simulink model "RLFactorySensorNoise"  (R2020b)
settings: Solver=VariableStepAuto  StartTime=0.0  StopTime=10.0  RelTol=1e-3
undefined symbols (not defined in the file): BLOCKEDTIMER, CUTOFF, DMAX, GOALSA, GOALSB, INITBX, INITBY, INTERFERENCEMAX, INTERFERENCEMIN, MAXVELOA, MAXVELOB, SAFETYDISTANCEA, SAFETYDISTANCEB, THRESHOLDA, THRESHOLDB, TSA, TSB, TSRL
libraries: rllib x1
(part 1 of 2)
settings Model: Creator=julius  LastModifiedBy=julius

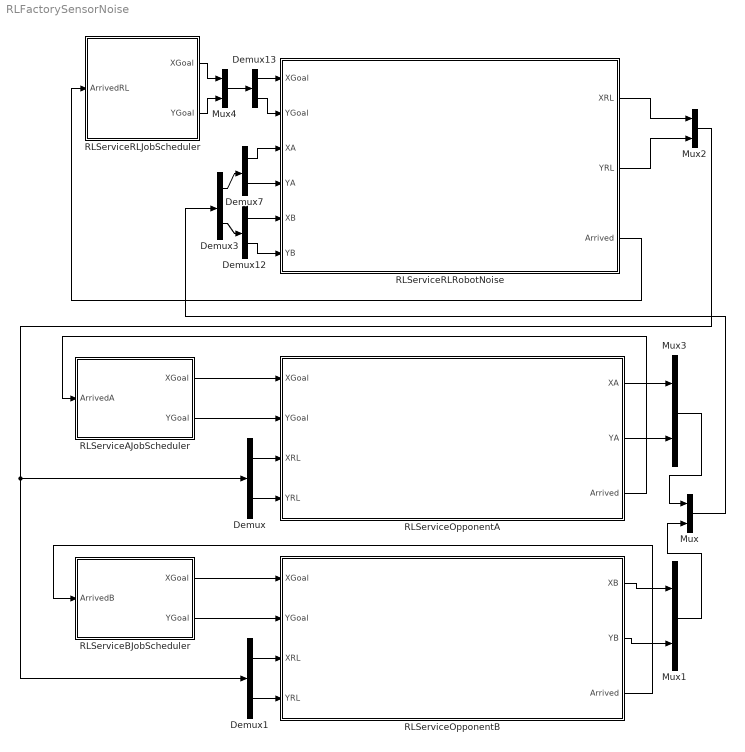
== system RLFactorySensorNoise ==
  Demux{,1,3,7,12..13} (6 alike) : Demux  Outputs=2
  Mux{,1..4} (5 alike) : Mux  Inputs=2
  RLServiceAJobScheduler : Subsystem
  RLServiceBJobScheduler : Subsystem
  RLServiceOpponentA : Subsystem
  RLServiceOpponentB : Subsystem
  RLServiceRLJobScheduler : Subsystem
  RLServiceRLRobotNoise : Subsystem
  wires:
  RLServiceRLJobScheduler/2(YGoal) -> Mux4/2
  RLServiceRLJobScheduler/1(XGoal) -> Mux4/1
  Mux4/1 -> Demux13/1
  Demux3/1 -> Demux7/1
  Demux3/2 -> Demux12/1
  Demux13/1 -> RLServiceRLRobotNoise/1(XGoal)
  Demux13/2 -> RLServiceRLRobotNoise/2(YGoal)
  Demux7/1 -> RLServiceRLRobotNoise/3(XA)
  Demux7/2 -> RLServiceRLRobotNoise/4(YA)
  Demux12/1 -> RLServiceRLRobotNoise/5(XB)
  Demux12/2 -> RLServiceRLRobotNoise/6(YB)
  RLServiceRLRobotNoise/3(Arrived) -> RLServiceRLJobScheduler/1(ArrivedRL)
  RLServiceRLRobotNoise/1(XRL) -> Mux2/1
  RLServiceRLRobotNoise/2(YRL) -> Mux2/2
  RLServiceOpponentB/3(Arrived) -> RLServiceBJobScheduler/1(ArrivedB)
  Demux1/2 -> RLServiceOpponentB/4(YRL)
  Demux/2 -> RLServiceOpponentA/4(YRL)
  Mux1/1 -> Mux/2
  RLServiceBJobScheduler/2(YGoal) -> RLServiceOpponentB/2(YGoal)
  RLServiceBJobScheduler/1(XGoal) -> RLServiceOpponentB/1(XGoal)
  RLServiceOpponentA/1(XA) -> Mux3/1
  RLServiceOpponentB/1(XB) -> Mux1/1
  Demux1/1 -> RLServiceOpponentB/3(XRL)
  Mux/1 -> Demux3/1
  RLServiceOpponentB/2(YB) -> Mux1/2
  RLServiceOpponentA/2(YA) -> Mux3/2
  RLServiceAJobScheduler/2(YGoal) -> RLServiceOpponentA/2(YGoal)
  RLServiceOpponentA/3(Arrived) -> RLServiceAJobScheduler/1(ArrivedA)
  Demux/1 -> RLServiceOpponentA/3(XRL)
  RLServiceAJobScheduler/1(XGoal) -> RLServiceOpponentA/1(XGoal)
  Mux3/1 -> Mux/1
  Mux2/1 -> Demux1/1, Demux/1

== system RLFactorySensorNoise/RLServiceAJobScheduler ==
  ArrivedA : Inport
  Constant1 : Constant  Value=GOALSA
  JobScheduler2 : MATLABSystem  System=JobScheduler  SimulateUsing=Interpreted execution
      mask Type: JobScheduler
      mask Display:
      | disp('JobScheduler');
      | port_label('input',1,'workstations');
      | port_label('input',2,'done');
      | port_label('output',1,'currentGoalX');
      | port_label('output',2,'currentGoalY');
  XGoal : Outport
  YGoal : Outport  Port=2
  wires:
  Constant1/1 -> JobScheduler2/1
  JobScheduler2/2 -> YGoal/1
  ArrivedA/1 -> JobScheduler2/2
  JobScheduler2/1 -> XGoal/1

== system RLFactorySensorNoise/RLServiceBJobScheduler ==
  ArrivedB : Inport
  Constant1 : Constant  Value=GOALSB
  JobScheduler2 : MATLABSystem  System=JobScheduler  SimulateUsing=Interpreted execution
      mask Type: JobScheduler
      mask Display:
      | disp('JobScheduler');
      | port_label('input',1,'workstations');
      | port_label('input',2,'done');
      | port_label('output',1,'currentGoalX');
      | port_label('output',2,'currentGoalY');
  XGoal : Outport
  YGoal : Outport  Port=2
  wires:
  Constant1/1 -> JobScheduler2/1
  JobScheduler2/2 -> YGoal/1
  ArrivedB/1 -> JobScheduler2/2
  JobScheduler2/1 -> XGoal/1

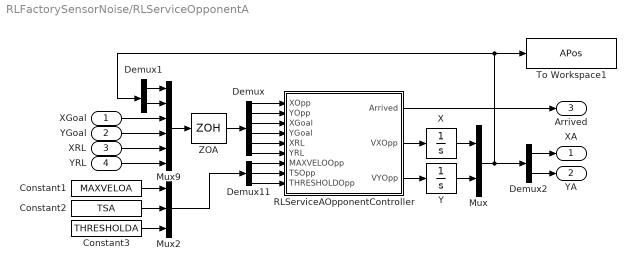
== system RLFactorySensorNoise/RLServiceOpponentA ==
  XGoal : Inport
  YGoal : Inport  Port=2
  XRL : Inport  Port=3
  YRL : Inport  Port=4
  Constant1 : Constant  Value=MAXVELOA
  Constant2 : Constant  Value=TSA
  Constant3 : Constant  Value=THRESHOLDA
  Demux : Demux  Outputs=6
  Demux1 : Demux  Outputs=2
  Demux11 : Demux  Outputs=3
  Demux2 : Demux  Outputs=2
  Mux : Mux  Inputs=2
  Mux2 : Mux  Inputs=3
  Mux9 : Mux  Inputs=6
  RLServiceAOpponentController : Subsystem
  To Workspace1 : ToWorkspace  VariableName=APos  SampleTime=0.25
  X : Integrator  InitialCondition=5
  Y : Integrator  InitialCondition=5
  ZOA : ZeroOrderHold  SampleTime=TSA
  XA : Outport
  YA : Outport  Port=2
  Arrived : Outport  Port=3
  wires:
  RLServiceAOpponentController/1(Arrived) -> Arrived/1
  Demux/4 -> RLServiceAOpponentController/4(YGoal)
  Demux/6 -> RLServiceAOpponentController/6(YRL)
  X/1 -> Mux/1
  YRL/1 -> Mux9/6
  Demux/5 -> RLServiceAOpponentController/5(XRL)
  YGoal/1 -> Mux9/4
  Demux/1 -> RLServiceAOpponentController/1(XOpp)
  Y/1 -> Mux/2
  Mux/1 -> Demux1/1, To Workspace1/1, Demux2/1
  Mux9/1 -> ZOA/1
  Demux/3 -> RLServiceAOpponentController/3(XGoal)
  Demux/2 -> RLServiceAOpponentController/2(YOpp)
  XRL/1 -> Mux9/5
  ZOA/1 -> Demux/1
  XGoal/1 -> Mux9/3
  Mux2/1 -> Demux11/1
  Demux1/1 -> Mux9/1
  Demux1/2 -> Mux9/2
  Constant2/1 -> Mux2/2
  Constant1/1 -> Mux2/1
  Constant3/1 -> Mux2/3
  Demux2/1 -> XA/1
  Demux2/2 -> YA/1
  RLServiceAOpponentController/3(VYOpp) -> Y/1
  RLServiceAOpponentController/2(VXOpp) -> X/1
  Demux11/1 -> RLServiceAOpponentController/7(MAXVELOOpp)
  Demux11/2 -> RLServiceAOpponentController/8(TSOpp)
  Demux11/3 -> RLServiceAOpponentController/9(THRESHOLDOpp)

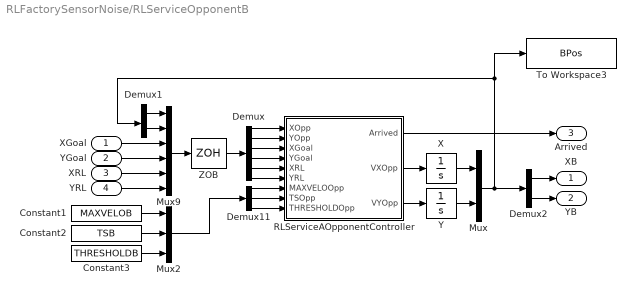
== system RLFactorySensorNoise/RLServiceOpponentB ==
  XGoal : Inport
  YGoal : Inport  Port=2
  XRL : Inport  Port=3
  YRL : Inport  Port=4
  Constant1 : Constant  Value=MAXVELOB
  Constant2 : Constant  Value=TSB
  Constant3 : Constant  Value=THRESHOLDB
  Demux : Demux  Outputs=6
  Demux1 : Demux  Outputs=2
  Demux11 : Demux  Outputs=3
  Demux2 : Demux  Outputs=2
  Mux : Mux  Inputs=2
  Mux2 : Mux  Inputs=3
  Mux9 : Mux  Inputs=6
  RLServiceAOpponentController : Subsystem
  To Workspace3 : ToWorkspace  VariableName=BPos  SampleTime=0.25
  X : Integrator  InitialCondition=randi(INITBX)
  Y : Integrator  InitialCondition=randi(INITBY)
  ZOB : ZeroOrderHold  SampleTime=TSB
  XB : Outport
  YB : Outport  Port=2
  Arrived : Outport  Port=3
  wires:
  RLServiceAOpponentController/3(VYOpp) -> Y/1
  XRL/1 -> Mux9/5
  Demux11/1 -> RLServiceAOpponentController/7(MAXVELOOpp)
  Constant2/1 -> Mux2/2
  RLServiceAOpponentController/2(VXOpp) -> X/1
  Mux9/1 -> ZOB/1
  Constant3/1 -> Mux2/3
  Demux1/2 -> Mux9/2
  Demux/1 -> RLServiceAOpponentController/1(XOpp)
  YGoal/1 -> Mux9/4
  Demux/4 -> RLServiceAOpponentController/4(YGoal)
  RLServiceAOpponentController/1(Arrived) -> Arrived/1
  X/1 -> Mux/1
  Mux/1 -> To Workspace3/1, Demux1/1, Demux2/1
  Demux/6 -> RLServiceAOpponentController/6(YRL)
  Demux/3 -> RLServiceAOpponentController/3(XGoal)
  Demux1/1 -> Mux9/1
  Demux11/2 -> RLServiceAOpponentController/8(TSOpp)
  Demux2/1 -> XB/1
  YRL/1 -> Mux9/6
  Demux/2 -> RLServiceAOpponentController/2(YOpp)
  Demux11/3 -> RLServiceAOpponentController/9(THRESHOLDOpp)
  ZOB/1 -> Demux/1
  Demux2/2 -> YB/1
  Mux2/1 -> Demux11/1
  Constant1/1 -> Mux2/1
  XGoal/1 -> Mux9/3
  Y/1 -> Mux/2
  Demux/5 -> RLServiceAOpponentController/5(XRL)

== system RLFactorySensorNoise/RLServiceRLJobScheduler ==
  ArrivedRL : Inport
  Constant : Constant  Value=[[-3;4],[5;5],[-5;-5],[5;2]]
  JobScheduler1 : MATLABSystem  System=JobScheduler  SimulateUsing=Interpreted execution
      mask Type: JobScheduler
      mask Display:
      | disp('JobScheduler');
      | port_label('input',1,'workstations');
      | port_label('input',2,'done');
      | port_label('output',1,'currentGoalX');
      | port_label('output',2,'currentGoalY');
  Mux2 : Mux  Inputs=2
  To Workspace2 : ToWorkspace  VariableName=Job  SampleTime=0.25
  XGoal : Outport
  YGoal : Outport  Port=2
  wires:
  Constant/1 -> JobScheduler1/1
  JobScheduler1/2 -> Mux2/2, YGoal/1
  ArrivedRL/1 -> JobScheduler1/2
  JobScheduler1/1 -> Mux2/1, XGoal/1
  Mux2/1 -> To Workspace2/1

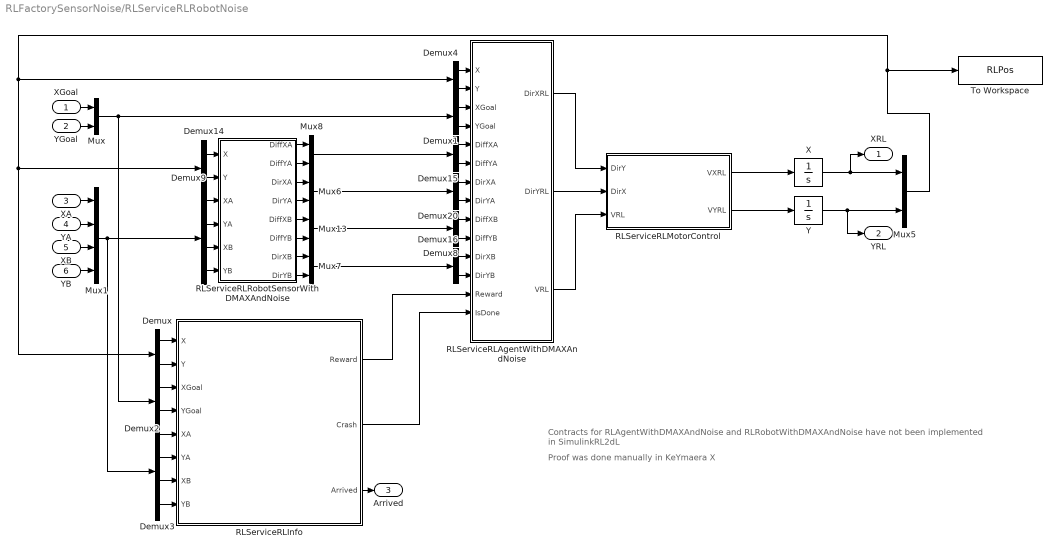
== system RLFactorySensorNoise/RLServiceRLRobotNoise ==
  note: Proof was done manually in KeYmaera X
  note: Contracts for RLAgentWithDMAXAndNoise and RLRobotWithDMAXAndNoise have not been implemented in SimulinkRL2dL
  XGoal : Inport
  YGoal : Inport  Port=2
  XA : Inport  Port=3
  YA : Inport  Port=4
  XB : Inport  Port=5
  YB : Inport  Port=6
  Demux{,1..2,4,8,14..16,20} (9 alike) : Demux  Outputs=2
  Demux3 : Demux
  Demux9 : Demux
  Mux{,5..8,13} (6 alike) : Mux  Inputs=2
  Mux1 : Mux
  RLServiceRLAgentWithDMAXAndNoise : Subsystem
  RLServiceRLInfo : Subsystem
  RLServiceRLMotorControl : Subsystem
  RLServiceRLRobotSensorWithDMAXAndNoise : Subsystem
  To Workspace : ToWorkspace  VariableName=RLPos  SampleTime=0.25
  X : Integrator  InitialCondition=-3
  Y : Integrator  InitialCondition=-5
  XRL : Outport
  YRL : Outport  Port=2
  Arrived : Outport  Port=3
  wires:
  XA/1 -> Mux1/1
  X/1 -> Mux5/1, XRL/1
  Mux13/1 -> Demux8/1
  Demux4/1 -> RLServiceRLAgentWithDMAXAndNoise/1(X)
  RLServiceRLRobotSensorWithDMAXAndNoise/5(DiffXB) -> Mux13/1
  Demux4/2 -> RLServiceRLAgentWithDMAXAndNoise/2(Y)
  Demux14/2 -> RLServiceRLRobotSensorWithDMAXAndNoise/2(Y)
  Demux15/1 -> RLServiceRLAgentWithDMAXAndNoise/5(DiffXA)
  RLServiceRLRobotSensorWithDMAXAndNoise/4(DirYA) -> Mux6/2
  XGoal/1 -> Mux/1
  Demux20/2 -> RLServiceRLAgentWithDMAXAndNoise/8(DirYA)
  RLServiceRLRobotSensorWithDMAXAndNoise/2(DiffYA) -> Mux8/2
  RLServiceRLRobotSensorWithDMAXAndNoise/7(DirXB) -> Mux7/1
  Mux/1 -> Demux2/1, Demux1/1
  Demux1/2 -> RLServiceRLAgentWithDMAXAndNoise/4(YGoal)
  Demux16/1 -> RLServiceRLAgentWithDMAXAndNoise/11(DirXB)
  RLServiceRLInfo/1(Reward) -> RLServiceRLAgentWithDMAXAndNoise/13(Reward)
  Demux15/2 -> RLServiceRLAgentWithDMAXAndNoise/6(DiffYA)
  Demux1/1 -> RLServiceRLAgentWithDMAXAndNoise/3(XGoal)
  Y/1 -> YRL/1, Mux5/2
  RLServiceRLRobotSensorWithDMAXAndNoise/3(DirXA) -> Mux6/1
  RLServiceRLAgentWithDMAXAndNoise/2(DirYRL) -> RLServiceRLMotorControl/2(DirX)
  Mux1/1 -> Demux3/1, Demux9/1
  Demux20/1 -> RLServiceRLAgentWithDMAXAndNoise/7(DirXA)
  RLServiceRLRobotSensorWithDMAXAndNoise/8(DirYB) -> Mux7/2
  Demux8/1 -> RLServiceRLAgentWithDMAXAndNoise/9(DiffXB)
  YB/1 -> Mux1/4
  YGoal/1 -> Mux/2
  Mux5/1 -> Demux4/1, Demux/1, Demux14/1, To Workspace/1
  Mux6/1 -> Demux20/1
  RLServiceRLAgentWithDMAXAndNoise/1(DirXRL) -> RLServiceRLMotorControl/1(DirY)
  RLServiceRLRobotSensorWithDMAXAndNoise/1(DiffXA) -> Mux8/1
  Mux7/1 -> Demux16/1
  XB/1 -> Mux1/3
  Demux16/2 -> RLServiceRLAgentWithDMAXAndNoise/12(DirYB)
  YA/1 -> Mux1/2
  Demux8/2 -> RLServiceRLAgentWithDMAXAndNoise/10(DiffYB)
  Mux8/1 -> Demux15/1
  Demux14/1 -> RLServiceRLRobotSensorWithDMAXAndNoise/1(X)
  RLServiceRLRobotSensorWithDMAXAndNoise/6(DiffYB) -> Mux13/2
  RLServiceRLAgentWithDMAXAndNoise/3(VRL) -> RLServiceRLMotorControl/3(VRL)
  RLServiceRLMotorControl/1(VXRL) -> X/1
  RLServiceRLMotorControl/2(VYRL) -> Y/1
  RLServiceRLInfo/2(Crash) -> RLServiceRLAgentWithDMAXAndNoise/14(IsDone)
  RLServiceRLInfo/3(Arrived) -> Arrived/1
  Demux9/1 -> RLServiceRLRobotSensorWithDMAXAndNoise/3(XA)
  Demux9/2 -> RLServiceRLRobotSensorWithDMAXAndNoise/4(YA)
  Demux9/3 -> RLServiceRLRobotSensorWithDMAXAndNoise/5(XB)
  Demux9/4 -> RLServiceRLRobotSensorWithDMAXAndNoise/6(YB)
  Demux/1 -> RLServiceRLInfo/1(X)
  Demux/2 -> RLServiceRLInfo/2(Y)
  Demux2/1 -> RLServiceRLInfo/3(XGoal)
  Demux2/2 -> RLServiceRLInfo/4(YGoal)
  Demux3/1 -> RLServiceRLInfo/5(XA)
  Demux3/2 -> RLServiceRLInfo/6(YA)
  Demux3/3 -> RLServiceRLInfo/7(XB)
  Demux3/4 -> RLServiceRLInfo/8(YB)

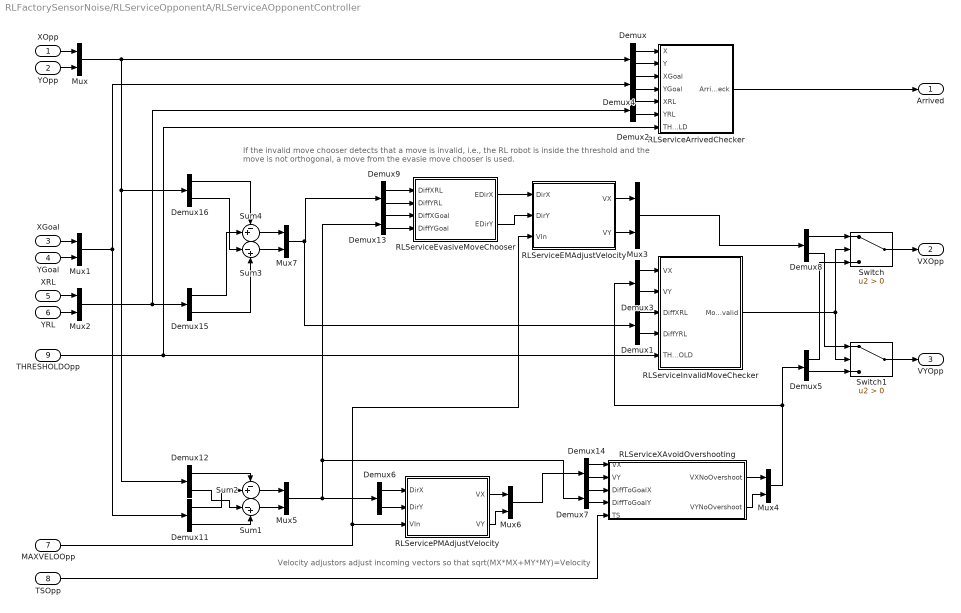
== system RLFactorySensorNoise/RLServiceOpponentA/RLServiceAOpponentController ==
  note: If the invalid move chooser detects that a move is invalid, i.e.,
      | the RL robot is inside the threshold and the move is not orthogonal, a move from the evasie move chooser is used.
  note: Velocity adjustors adjust incoming vectors so that sqrt(MX*MX+MY*MY)=Velocity
  XOpp : Inport
  YOpp : Inport  Port=2
  XGoal : Inport  Port=3
  YGoal : Inport  Port=4
  XRL : Inport  Port=5
  YRL : Inport  Port=6
  MAXVELOOpp : Inport  Port=7
  TSOpp : Inport  Port=8
  THRESHOLDOpp : Inport  Port=9
  Demux{,1..9,11..16} (16 alike) : Demux  Outputs=2
  Mux{,1..7} (8 alike) : Mux  Inputs=2
  RLServiceArrivedChecker : Subsystem
  RLServiceEMAdjustVelocity : Subsystem
  RLServiceEvasiveMoveChooser : Subsystem
  RLServiceInvalidMoveChecker : Subsystem
  RLServicePMAdjustVelocity : Subsystem
  RLServiceXAvoidOvershooting : Subsystem
  Sum1 : Sum  Inputs=|-+
  Sum2 : Sum  Inputs=-+|
  Sum3 : Sum  Inputs=|-+
  Sum4 : Sum  Inputs=-+|
  Switch : Switch  Criteria=u2 > Threshold
  Switch1 : Switch  Criteria=u2 > Threshold
  Arrived : Outport
  VXOpp : Outport  Port=2
  VYOpp : Outport  Port=3
  wires:
  XGoal/1 -> Mux1/1
  YGoal/1 -> Mux1/2
  RLServiceArrivedChecker/1(ArrivedCheck) -> Arrived/1
  Demux/1 -> RLServiceArrivedChecker/1(X)
  Demux/2 -> RLServiceArrivedChecker/2(Y)
  Demux4/1 -> RLServiceArrivedChecker/3(XGoal)
  Demux4/2 -> RLServiceArrivedChecker/4(YGoal)
  XOpp/1 -> Mux/1
  YOpp/1 -> Mux/2
  XRL/1 -> Mux2/1
  YRL/1 -> Mux2/2
  Demux3/1 -> RLServiceInvalidMoveChecker/1(VX)
  Demux8/1 -> Switch/1
  Demux5/2 -> Switch1/3
  Demux8/2 -> Switch1/1
  THRESHOLDOpp/1 -> RLServiceArrivedChecker/7(THRESHOLD), RLServiceInvalidMoveChecker/5(THRESHOLD)
  Demux3/2 -> RLServiceInvalidMoveChecker/2(VY)
  Demux5/1 -> Switch/3
  RLServiceInvalidMoveChecker/1(MoveInvalid) -> Switch/2, Switch1/2
  Switch/1 -> VXOpp/1
  Switch1/1 -> VYOpp/1
  Mux5/1 -> Demux6/1, Demux7/1, Demux13/1
  Demux6/2 -> RLServicePMAdjustVelocity/2(DirY)
  Mux1/1 -> Demux4/1, Demux11/1
  TSOpp/1 -> RLServiceXAvoidOvershooting/5(TS)
  MAXVELOOpp/1 -> RLServiceEMAdjustVelocity/3(VIn), RLServicePMAdjustVelocity/3(VIn)
  RLServicePMAdjustVelocity/1(VX) -> Mux6/1
  RLServicePMAdjustVelocity/2(VY) -> Mux6/2
  RLServiceEvasiveMoveChooser/1(EDirX) -> RLServiceEMAdjustVelocity/1(DirX)
  RLServiceEvasiveMoveChooser/2(EDirY) -> RLServiceEMAdjustVelocity/2(DirY)
  RLServiceEMAdjustVelocity/1(VX) -> Mux3/1
  RLServiceEMAdjustVelocity/2(VY) -> Mux3/2
  Mux3/1 -> Demux8/1
  RLServiceXAvoidOvershooting/1(VXNoOvershoot) -> Mux4/1
  RLServiceXAvoidOvershooting/2(VYNoOvershoot) -> Mux4/2
  Mux4/1 -> Demux5/1, Demux3/1
  Sum2/1 -> Mux5/1
  Sum1/1 -> Mux5/2
  Demux6/1 -> RLServicePMAdjustVelocity/1(DirX)
  Demux7/1 -> RLServiceXAvoidOvershooting/3(DiffToGoalX)
  Demux7/2 -> RLServiceXAvoidOvershooting/4(DiffToGoalY)
  Demux13/1 -> RLServiceEvasiveMoveChooser/3(DiffXGoal)
  Demux13/2 -> RLServiceEvasiveMoveChooser/4(DiffYGoal)
  Demux11/1 -> Sum2/2
  Demux12/2 -> Sum1/1
  Demux11/2 -> Sum1/2
  Demux12/1 -> Sum2/1
  Demux14/1 -> RLServiceXAvoidOvershooting/1(VX)
  Demux14/2 -> RLServiceXAvoidOvershooting/2(VY)
  Mux6/1 -> Demux14/1
  Sum3/1 -> Mux7/2
  Demux16/1 -> Sum4/1
  Sum4/1 -> Mux7/1
  Mux/1 -> Demux12/1, Demux16/1, Demux/1
  Mux2/1 -> Demux2/1, Demux15/1
  Demux15/2 -> Sum3/2
  Demux15/1 -> Sum4/2
  Demux16/2 -> Sum3/1
  Demux9/1 -> RLServiceEvasiveMoveChooser/1(DiffXRL)
  Demux9/2 -> RLServiceEvasiveMoveChooser/2(DiffYRL)
  Mux7/1 -> Demux1/1, Demux9/1
  Demux1/1 -> RLServiceInvalidMoveChecker/3(DiffXRL)
  Demux1/2 -> RLServiceInvalidMoveChecker/4(DiffYRL)
  Demux2/2 -> RLServiceArrivedChecker/6(YRL)
  Demux2/1 -> RLServiceArrivedChecker/5(XRL)

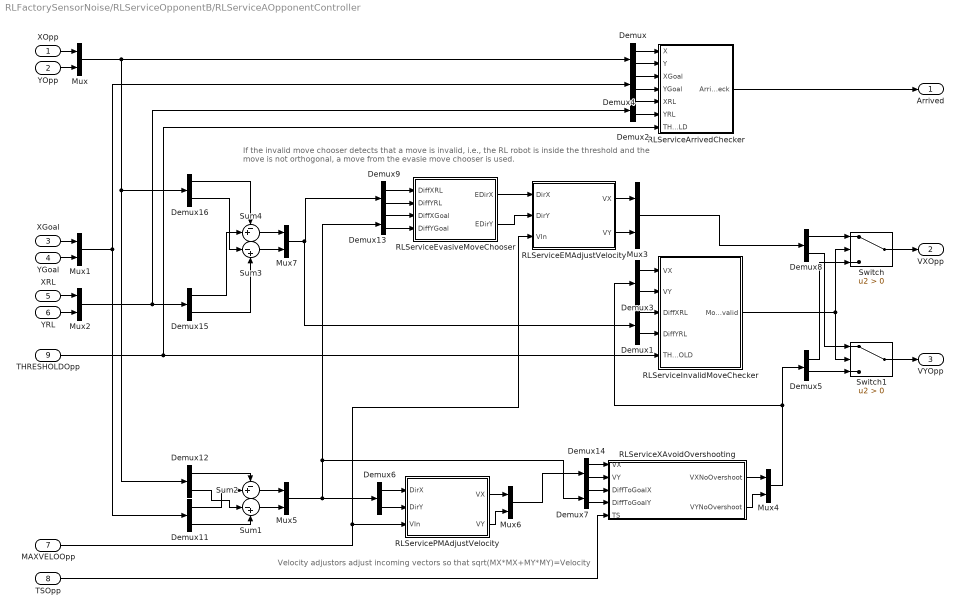
== system RLFactorySensorNoise/RLServiceOpponentB/RLServiceAOpponentController ==
  note: If the invalid move chooser detects that a move is invalid, i.e.,
      | the RL robot is inside the threshold and the move is not orthogonal, a move from the evasie move chooser is used.
  note: Velocity adjustors adjust incoming vectors so that sqrt(MX*MX+MY*MY)=Velocity
  XOpp : Inport
  YOpp : Inport  Port=2
  XGoal : Inport  Port=3
  YGoal : Inport  Port=4
  XRL : Inport  Port=5
  YRL : Inport  Port=6
  MAXVELOOpp : Inport  Port=7
  TSOpp : Inport  Port=8
  THRESHOLDOpp : Inport  Port=9
  Demux{,1..9,11..16} (16 alike) : Demux  Outputs=2
  Mux{,1..7} (8 alike) : Mux  Inputs=2
  RLServiceArrivedChecker : Subsystem
  RLServiceEMAdjustVelocity : Subsystem
  RLServiceEvasiveMoveChooser : Subsystem
  RLServiceInvalidMoveChecker : Subsystem
  RLServicePMAdjustVelocity : Subsystem
  RLServiceXAvoidOvershooting : Subsystem
  Sum1 : Sum  Inputs=|-+
  Sum2 : Sum  Inputs=-+|
  Sum3 : Sum  Inputs=|-+
  Sum4 : Sum  Inputs=-+|
  Switch : Switch  Criteria=u2 > Threshold
  Switch1 : Switch  Criteria=u2 > Threshold
  Arrived : Outport
  VXOpp : Outport  Port=2
  VYOpp : Outport  Port=3
  wires:
  XGoal/1 -> Mux1/1
  YGoal/1 -> Mux1/2
  RLServiceArrivedChecker/1(ArrivedCheck) -> Arrived/1
  Demux/1 -> RLServiceArrivedChecker/1(X)
  Demux/2 -> RLServiceArrivedChecker/2(Y)
  Demux4/1 -> RLServiceArrivedChecker/3(XGoal)
  Demux4/2 -> RLServiceArrivedChecker/4(YGoal)
  XOpp/1 -> Mux/1
  YOpp/1 -> Mux/2
  XRL/1 -> Mux2/1
  YRL/1 -> Mux2/2
  Demux3/1 -> RLServiceInvalidMoveChecker/1(VX)
  Demux8/1 -> Switch/1
  Demux5/2 -> Switch1/3
  Demux8/2 -> Switch1/1
  THRESHOLDOpp/1 -> RLServiceArrivedChecker/7(THRESHOLD), RLServiceInvalidMoveChecker/5(THRESHOLD)
  Demux3/2 -> RLServiceInvalidMoveChecker/2(VY)
  Demux5/1 -> Switch/3
  RLServiceInvalidMoveChecker/1(MoveInvalid) -> Switch/2, Switch1/2
  Switch/1 -> VXOpp/1
  Switch1/1 -> VYOpp/1
  Mux5/1 -> Demux6/1, Demux7/1, Demux13/1
  Demux6/2 -> RLServicePMAdjustVelocity/2(DirY)
  Mux1/1 -> Demux4/1, Demux11/1
  TSOpp/1 -> RLServiceXAvoidOvershooting/5(TS)
  MAXVELOOpp/1 -> RLServiceEMAdjustVelocity/3(VIn), RLServicePMAdjustVelocity/3(VIn)
  RLServicePMAdjustVelocity/1(VX) -> Mux6/1
  RLServicePMAdjustVelocity/2(VY) -> Mux6/2
  RLServiceEvasiveMoveChooser/1(EDirX) -> RLServiceEMAdjustVelocity/1(DirX)
  RLServiceEvasiveMoveChooser/2(EDirY) -> RLServiceEMAdjustVelocity/2(DirY)
  RLServiceEMAdjustVelocity/1(VX) -> Mux3/1
  RLServiceEMAdjustVelocity/2(VY) -> Mux3/2
  Mux3/1 -> Demux8/1
  RLServiceXAvoidOvershooting/1(VXNoOvershoot) -> Mux4/1
  RLServiceXAvoidOvershooting/2(VYNoOvershoot) -> Mux4/2
  Mux4/1 -> Demux5/1, Demux3/1
  Sum2/1 -> Mux5/1
  Sum1/1 -> Mux5/2
  Demux6/1 -> RLServicePMAdjustVelocity/1(DirX)
  Demux7/1 -> RLServiceXAvoidOvershooting/3(DiffToGoalX)
  Demux7/2 -> RLServiceXAvoidOvershooting/4(DiffToGoalY)
  Demux13/1 -> RLServiceEvasiveMoveChooser/3(DiffXGoal)
  Demux13/2 -> RLServiceEvasiveMoveChooser/4(DiffYGoal)
  Demux11/1 -> Sum2/2
  Demux12/2 -> Sum1/1
  Demux11/2 -> Sum1/2
  Demux12/1 -> Sum2/1
  Demux14/1 -> RLServiceXAvoidOvershooting/1(VX)
  Demux14/2 -> RLServiceXAvoidOvershooting/2(VY)
  Mux6/1 -> Demux14/1
  Sum3/1 -> Mux7/2
  Demux16/1 -> Sum4/1
  Sum4/1 -> Mux7/1
  Mux/1 -> Demux12/1, Demux16/1, Demux/1
  Mux2/1 -> Demux2/1, Demux15/1
  Demux15/2 -> Sum3/2
  Demux15/1 -> Sum4/2
  Demux16/2 -> Sum3/1
  Demux9/1 -> RLServiceEvasiveMoveChooser/1(DiffXRL)
  Demux9/2 -> RLServiceEvasiveMoveChooser/2(DiffYRL)
  Mux7/1 -> Demux1/1, Demux9/1
  Demux1/1 -> RLServiceInvalidMoveChecker/3(DiffXRL)
  Demux1/2 -> RLServiceInvalidMoveChecker/4(DiffYRL)
  Demux2/2 -> RLServiceArrivedChecker/6(YRL)
  Demux2/1 -> RLServiceArrivedChecker/5(XRL)

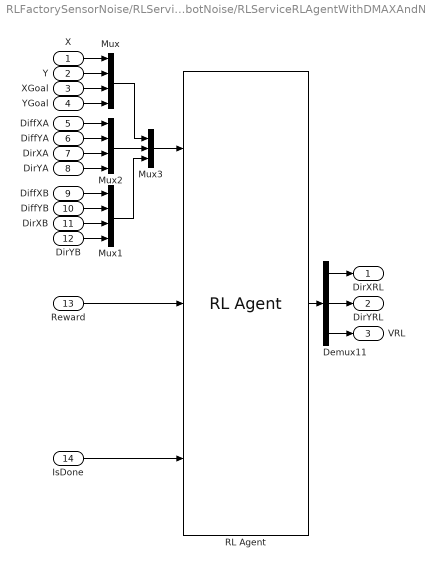
== system RLFactorySensorNoise/RLServiceRLRobotNoise/RLServiceRLAgentWithDMAXAndNoise ==
  X : Inport
  Y : Inport  Port=2
  XGoal : Inport  Port=3
  YGoal : Inport  Port=4
  DiffXA : Inport  Port=5
  DiffYA : Inport  Port=6
  DirXA : Inport  Port=7
  DirYA : Inport  Port=8
  DiffXB : Inport  Port=9
  DiffYB : Inport  Port=10
  DirXB : Inport  Port=11
  DirYB : Inport  Port=12
  Reward : Inport  Port=13
  IsDone : Inport  Port=14
  Demux11 : Demux  Outputs=3
  Mux : Mux
  Mux1 : Mux
  Mux2 : Mux
  Mux3 : Mux  Inputs=3
  RL Agent : rllib/RL Agent  Agent=qAgent  ProvideReward=on  ProvideIsDone=on  ProvideCumRwd=off  TreatAsDirectFeedthrough=on  CollectLoggedSignals=on  CollectModelStates=on
  DirXRL : Outport
  DirYRL : Outport  Port=2
  VRL : Outport  Port=3
  wires:
  IsDone/1 -> RL Agent/3
  Demux11/1 -> DirXRL/1
  Reward/1 -> RL Agent/2
  DirXA/1 -> Mux2/3
  YGoal/1 -> Mux/4
  DiffXA/1 -> Mux2/1
  X/1 -> Mux/1
  XGoal/1 -> Mux/3
  DirYA/1 -> Mux2/4
  DiffYA/1 -> Mux2/2
  Y/1 -> Mux/2
  DiffXB/1 -> Mux1/1
  DiffYB/1 -> Mux1/2
  DirXB/1 -> Mux1/3
  DirYB/1 -> Mux1/4
  Mux2/1 -> Mux3/2
  Mux3/1 -> RL Agent/1
  Mux/1 -> Mux3/1
  Mux1/1 -> Mux3/3
  RL Agent/1 -> Demux11/1
  Demux11/2 -> DirYRL/1
  Demux11/3 -> VRL/1

== system RLFactorySensorNoise/RLServiceRLRobotNoise/RLServiceRLInfo ==
  X : Inport
  Y : Inport  Port=2
  XGoal : Inport  Port=3
  YGoal : Inport  Port=4
  XA : Inport  Port=5
  YA : Inport  Port=6
  XB : Inport  Port=7
  YB : Inport  Port=8
  RLServiceCrashDetector : Subsystem
  RLServiceGoalTracker : Subsystem
  RLServiceReward : Subsystem
  To Workspace1 : ToWorkspace  VariableName=Crash  SampleTime=0.25
  To Workspace2 : ToWorkspace  VariableName=BelowThresh  SampleTime=0.25
  Reward : Outport
  Crash : Outport  Port=2
  Arrived : Outport  Port=3
  wires:
  YB/1 -> RLServiceCrashDetector/6(YB)
  YGoal/1 -> RLServiceGoalTracker/4(YGoal)
  XA/1 -> RLServiceCrashDetector/3(XA)
  RLServiceGoalTracker/2(Arrived) -> Arrived/1, RLServiceReward/2(Arrived)
  Y/1 -> RLServiceGoalTracker/2(Y), RLServiceCrashDetector/2(Y)
  XGoal/1 -> RLServiceGoalTracker/3(XGoal)
  XB/1 -> RLServiceCrashDetector/5(XB)
  RLServiceReward/1(Reward) -> Reward/1
  YA/1 -> RLServiceCrashDetector/4(YA)
  X/1 -> RLServiceGoalTracker/1(X), RLServiceCrashDetector/1(X)
  RLServiceGoalTracker/1(Dist) -> RLServiceReward/1(DistGoal)
  RLServiceCrashDetector/2(Crash) -> RLServiceReward/3(Crash), Crash/1, To Workspace1/1
  RLServiceCrashDetector/1(BelowThreshold) -> To Workspace2/1, RLServiceReward/4(BelowThreshold)

== system RLFactorySensorNoise/RLServiceRLRobotNoise/RLServiceRLMotorControl ==
  DirY : Inport
  DirX : Inport  Port=2
  VRL : Inport  Port=3
  RLServiceRLAdjustVelocity : Subsystem
  VXRL : Outport
  VYRL : Outport  Port=2
  wires:
  RLServiceRLAdjustVelocity/1(VX) -> VXRL/1
  RLServiceRLAdjustVelocity/2(VY) -> VYRL/1
  DirY/1 -> RLServiceRLAdjustVelocity/1(DirX)
  DirX/1 -> RLServiceRLAdjustVelocity/2(DirY)
  VRL/1 -> RLServiceRLAdjustVelocity/3(VIn)

== system RLFactorySensorNoise/RLServiceRLRobotNoise/RLServiceRLRobotSensorWithDMAXAndNoise ==
  X : Inport
  Y : Inport  Port=2
  XA : Inport  Port=3
  YA : Inport  Port=4
  XB : Inport  Port=5
  YB : Inport  Port=6
  RLServiceARobotSensorSubsystemWithDMAXAndNoise : Subsystem
  RLServiceBRobotSensorSubsystemWithDMAXAndNoise : Subsystem
  DiffXA : Outport
  DiffYA : Outport  Port=2
  DirXA : Outport  Port=3
  DirYA : Outport  Port=4
  DiffXB : Outport  Port=5
  DiffYB : Outport  Port=6
  DirXB : Outport  Port=7
  DirYB : Outport  Port=8
  wires:
  RLServiceBRobotSensorSubsystemWithDMAXAndNoise/3(DirX) -> DirXB/1
  YB/1 -> RLServiceBRobotSensorSubsystemWithDMAXAndNoise/4(YOpp)
  XB/1 -> RLServiceBRobotSensorSubsystemWithDMAXAndNoise/3(XOpp)
  RLServiceARobotSensorSubsystemWithDMAXAndNoise/4(DirY) -> DirYA/1
  X/1 -> RLServiceBRobotSensorSubsystemWithDMAXAndNoise/1(XRL), RLServiceARobotSensorSubsystemWithDMAXAndNoise/1(XRL)
  RLServiceBRobotSensorSubsystemWithDMAXAndNoise/4(DirY) -> DirYB/1
  Y/1 -> RLServiceBRobotSensorSubsystemWithDMAXAndNoise/2(YRL), RLServiceARobotSensorSubsystemWithDMAXAndNoise/2(YRL)
  RLServiceBRobotSensorSubsystemWithDMAXAndNoise/2(DiffY) -> DiffYB/1
  RLServiceARobotSensorSubsystemWithDMAXAndNoise/3(DirX) -> DirXA/1
  RLServiceBRobotSensorSubsystemWithDMAXAndNoise/1(DiffX) -> DiffXB/1
  XA/1 -> RLServiceARobotSensorSubsystemWithDMAXAndNoise/3(XOpp)
  YA/1 -> RLServiceARobotSensorSubsystemWithDMAXAndNoise/4(YOpp)
  RLServiceARobotSensorSubsystemWithDMAXAndNoise/1(DiffX) -> DiffXA/1
  RLServiceARobotSensorSubsystemWithDMAXAndNoise/2(DiffY) -> DiffYA/1

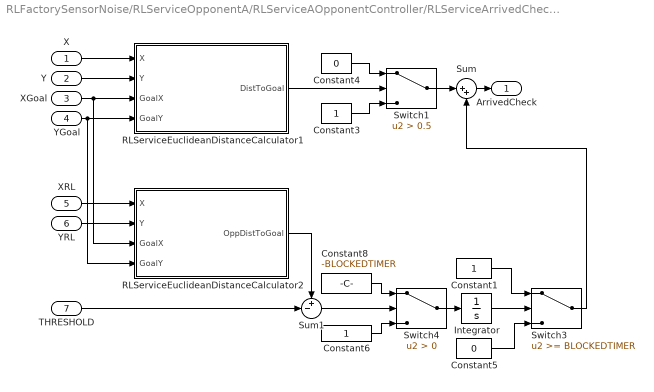
== system RLFactorySensorNoise/RLServiceOpponentA/RLServiceAOpponentController/RLServiceArrivedChecker ==
  X : Inport
  Y : Inport  Port=2
  XGoal : Inport  Port=3
  YGoal : Inport  Port=4
  XRL : Inport  Port=5
  YRL : Inport  Port=6
  THRESHOLD : Inport  Port=7
  Constant1 : Constant
  Constant3 : Constant
  Constant4 : Constant  Value=0
  Constant5 : Constant  Value=0
  Constant6 : Constant
  Constant8 : Constant  Value=-BLOCKEDTIMER
  Integrator : Integrator  LimitOutput=on  UpperSaturationLimit=BLOCKEDTIMER  LowerSaturationLimit=0
  RLServiceEuclideanDistanceCalculator1 : Subsystem
  RLServiceEuclideanDistanceCalculator2 : Subsystem
  Sum : Sum  Inputs=|++
  Sum1 : Sum  Inputs=+-|
  Switch1 : Switch  Criteria=u2 > Threshold  Threshold=0.5
  Switch3 : Switch  Threshold=BLOCKEDTIMER
  Switch4 : Switch  Criteria=u2 > Threshold
  ArrivedCheck : Outport
  wires:
  RLServiceEuclideanDistanceCalculator1/1(DistToGoal) -> Switch1/2
  X/1 -> RLServiceEuclideanDistanceCalculator1/1(X)
  Switch1/1 -> Sum/1
  Constant3/1 -> Switch1/3
  Y/1 -> RLServiceEuclideanDistanceCalculator1/2(Y)
  Constant4/1 -> Switch1/1
  Sum/1 -> ArrivedCheck/1
  Switch3/1 -> Sum/2
  Integrator/1 -> Switch3/2
  Constant5/1 -> Switch3/3
  XRL/1 -> RLServiceEuclideanDistanceCalculator2/1(X)
  YRL/1 -> RLServiceEuclideanDistanceCalculator2/2(Y)
  XGoal/1 -> RLServiceEuclideanDistanceCalculator2/3(GoalX), RLServiceEuclideanDistanceCalculator1/3(GoalX)
  YGoal/1 -> RLServiceEuclideanDistanceCalculator2/4(GoalY), RLServiceEuclideanDistanceCalculator1/4(GoalY)
  RLServiceEuclideanDistanceCalculator2/1(OppDistToGoal) -> Sum1/1
  Constant8/1 -> Switch4/1
  Constant6/1 -> Switch4/3
  THRESHOLD/1 -> Sum1/2
  Sum1/1 -> Switch4/2
  Switch4/1 -> Integrator/1
  Constant1/1 -> Switch3/1

== system RLFactorySensorNoise/RLServiceOpponentA/RLServiceAOpponentController/RLServiceEMAdjustVelocity ==
  DirX : Inport
  DirY : Inport  Port=2
  VIn : Inport  Port=3
  Constant : Constant
  Demux1 : Demux  Outputs=2
  Divide : Product  Inputs=*/
  Divide1 : Product  Inputs=*/
  Mux : Mux  Inputs=2
  Product : Product
  Product3 : Product
  Sqrt1 : Sqrt  SaturateOnIntegerOverflow=on
  Square : Math  Operator=square  SaturateOnIntegerOverflow=on
  Square1 : Math  Operator=square  SaturateOnIntegerOverflow=on
  Sum : Sum  Inputs=+|+
  Switch : Switch  Criteria=u2 > Threshold
  VX : Outport
  VY : Outport  Port=2
  wires:
  Product/1 -> VX/1
  DirY/1 -> Square1/1, Mux/2
  Mux/1 -> Demux1/1
  Divide1/1 -> Product3/1
  Constant/1 -> Switch/3
  Square1/1 -> Sum/2
  Switch/1 -> Divide1/2, Divide/2
  VIn/1 -> Product/2, Product3/2
  Sum/1 -> Sqrt1/1
  Square/1 -> Sum/1
  Sqrt1/1 -> Switch/2, Switch/1
  Product3/1 -> VY/1
  Demux1/2 -> Divide1/1
  DirX/1 -> Square/1, Mux/1
  Demux1/1 -> Divide/1
  Divide/1 -> Product/1

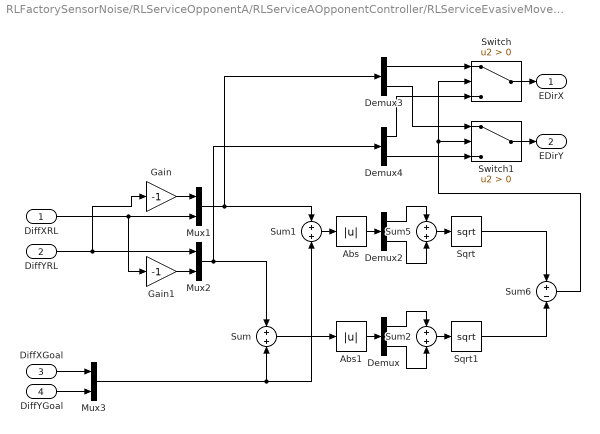
== system RLFactorySensorNoise/RLServiceOpponentA/RLServiceAOpponentController/RLServiceEvasiveMoveChooser ==
  DiffXRL : Inport
  DiffYRL : Inport  Port=2
  DiffXGoal : Inport  Port=3
  DiffYGoal : Inport  Port=4
  Abs : Abs
  Abs1 : Abs
  Demux{,2..4} (4 alike) : Demux  Outputs=2
  Gain : Gain  Gain=-1
  Gain1 : Gain  Gain=-1
  Mux1 : Mux  Inputs=2
  Mux2 : Mux  Inputs=2
  Mux3 : Mux  Inputs=2
  Sqrt : Sqrt  SaturateOnIntegerOverflow=on
  Sqrt1 : Sqrt  SaturateOnIntegerOverflow=on
  Sum{,1..2,5} (4 alike) : Sum  Inputs=+|+
  Sum6 : Sum  Inputs=+|-
  Switch : Switch  Criteria=u2 > Threshold
  Switch1 : Switch  Criteria=u2 > Threshold
  EDirX : Outport
  EDirY : Outport  Port=2
  wires:
  Gain/1 -> Mux1/1
  DiffXRL/1 -> Gain1/1, Mux1/2
  Gain1/1 -> Mux2/2
  DiffXGoal/1 -> Mux3/1
  DiffYGoal/1 -> Mux3/2
  Mux3/1 -> Sum/2, Sum1/2
  Mux2/1 -> Sum/1, Demux4/1
  Mux1/1 -> Demux3/1, Sum1/1
  Sum1/1 -> Abs/1
  Sum/1 -> Abs1/1
  Abs1/1 -> Demux/1
  Demux/1 -> Sum2/1
  Demux/2 -> Sum2/2
  Demux2/2 -> Sum5/2
  Demux2/1 -> Sum5/1
  Abs/1 -> Demux2/1
  Sum5/1 -> Sqrt/1
  Sum2/1 -> Sqrt1/1
  Sqrt/1 -> Sum6/1
  Sqrt1/1 -> Sum6/2
  Sum6/1 -> Switch/2, Switch1/2
  Demux3/1 -> Switch/1
  Demux3/2 -> Switch1/1
  Demux4/1 -> Switch/3
  Demux4/2 -> Switch1/3
  Switch/1 -> EDirX/1
  Switch1/1 -> EDirY/1
  DiffYRL/1 -> Mux2/1, Gain/1

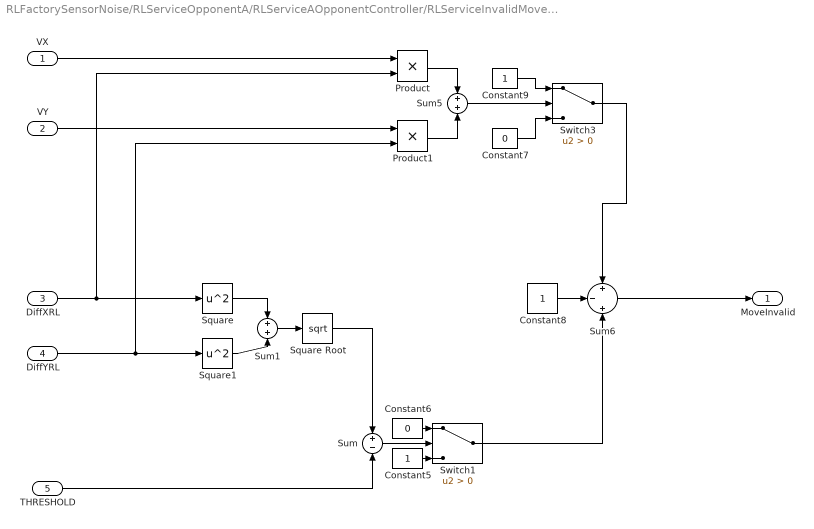
== system RLFactorySensorNoise/RLServiceOpponentA/RLServiceAOpponentController/RLServiceInvalidMoveChecker ==
  VX : Inport
  VY : Inport  Port=2
  DiffXRL : Inport  Port=3
  DiffYRL : Inport  Port=4
  THRESHOLD : Inport  Port=5
  Constant5 : Constant
  Constant6 : Constant  Value=0
  Constant7 : Constant  Value=0
  Constant8 : Constant
  Constant9 : Constant
  Product : Product
  Product1 : Product
  Square : Math  Operator=square  SaturateOnIntegerOverflow=on
  Square Root : Sqrt  SaturateOnIntegerOverflow=on
  Square1 : Math  Operator=square  SaturateOnIntegerOverflow=on
  Sum : Sum  Inputs=+|-
  Sum1 : Sum
  Sum5 : Sum  Inputs=+|+
  Sum6 : Sum  Inputs=+|-|+
  Switch1 : Switch  Criteria=u2 > Threshold
  Switch3 : Switch  Criteria=u2 > Threshold
  MoveInvalid : Outport
  wires:
  Product1/1 -> Sum5/2
  Sum5/1 -> Switch3/2
  Product/1 -> Sum5/1
  Sum6/1 -> MoveInvalid/1
  Switch3/1 -> Sum6/1
  Constant9/1 -> Switch3/1
  VY/1 -> Product1/1
  VX/1 -> Product/1
  Constant8/1 -> Sum6/2
  Constant7/1 -> Switch3/3
  THRESHOLD/1 -> Sum/2
  Sum/1 -> Switch1/2
  Constant5/1 -> Switch1/3
  Constant6/1 -> Switch1/1
  Switch1/1 -> Sum6/3
  DiffYRL/1 -> Square1/1, Product1/2
  DiffXRL/1 -> Product/2, Square/1
  Square1/1 -> Sum1/2
  Sum1/1 -> Square Root/1
  Square/1 -> Sum1/1
  Square Root/1 -> Sum/1

== system RLFactorySensorNoise/RLServiceOpponentA/RLServiceAOpponentController/RLServicePMAdjustVelocity ==
  DirX : Inport
  DirY : Inport  Port=2
  VIn : Inport  Port=3
  Constant : Constant
  Demux1 : Demux  Outputs=2
  Divide : Product  Inputs=*/
  Divide1 : Product  Inputs=*/
  Mux : Mux  Inputs=2
  Product : Product
  Product3 : Product
  Sqrt1 : Sqrt  SaturateOnIntegerOverflow=on
  Square : Math  Operator=square  SaturateOnIntegerOverflow=on
  Square1 : Math  Operator=square  SaturateOnIntegerOverflow=on
  Sum : Sum  Inputs=+|+
  Switch : Switch  Criteria=u2 > Threshold
  VX : Outport
  VY : Outport  Port=2
  wires:
  VIn/1 -> Product/2, Product3/2
  DirX/1 -> Square/1, Mux/1
  DirY/1 -> Square1/1, Mux/2
  Divide1/1 -> Product3/1
  Divide/1 -> Product/1
  Switch/1 -> Divide1/2, Divide/2
  Constant/1 -> Switch/3
  Mux/1 -> Demux1/1
  Demux1/2 -> Divide1/1
  Square1/1 -> Sum/2
  Sum/1 -> Sqrt1/1
  Demux1/1 -> Divide/1
  Product/1 -> VX/1
  Sqrt1/1 -> Switch/2, Switch/1
  Product3/1 -> VY/1
  Square/1 -> Sum/1

== system RLFactorySensorNoise/RLServiceOpponentA/RLServiceAOpponentController/RLServiceXAvoidOvershooting ==
  VX : Inport
  VY : Inport  Port=2
  DiffToGoalX : Inport  Port=3
  DiffToGoalY : Inport  Port=4
  TS : Inport  Port=5
  Abs{1..4} (4 alike) : Abs
  Divide : Product  Inputs=*/
  Divide1 : Product  Inputs=*/
  Product : Product
  Product1 : Product
  Sum1 : Sum  Inputs=-|+
  Sum2 : Sum  Inputs=-|+
  Switch : Switch  Criteria=u2 > Threshold
  Switch1 : Switch  Criteria=u2 > Threshold
  VXNoOvershoot : Outport
  VYNoOvershoot : Outport  Port=2
  wires:
  Abs1/1 -> Sum1/2
  Switch/1 -> VXNoOvershoot/1
  Product/1 -> Abs2/1
  Abs2/1 -> Sum1/1
  DiffToGoalX/1 -> Divide/1, Abs1/1
  Sum1/1 -> Switch/2
  VX/1 -> Product/1, Switch/1
  Divide/1 -> Switch/3
  VY/1 -> Product1/1, Switch1/1
  Sum2/1 -> Switch1/2
  Abs4/1 -> Sum2/1
  Product1/1 -> Abs4/1
  Divide1/1 -> Switch1/3
  TS/1 -> Divide1/2, Product1/2, Divide/2, Product/2
  Abs3/1 -> Sum2/2
  Switch1/1 -> VYNoOvershoot/1
  DiffToGoalY/1 -> Divide1/1, Abs3/1

== system RLFactorySensorNoise/RLServiceOpponentB/RLServiceAOpponentController/RLServiceArrivedChecker ==
  X : Inport
  Y : Inport  Port=2
  XGoal : Inport  Port=3
  YGoal : Inport  Port=4
  XRL : Inport  Port=5
  YRL : Inport  Port=6
  THRESHOLD : Inport  Port=7
  Constant1 : Constant
  Constant3 : Constant
  Constant4 : Constant  Value=0
  Constant5 : Constant  Value=0
  Constant6 : Constant
  Constant8 : Constant  Value=-BLOCKEDTIMER
  Integrator : Integrator  LimitOutput=on  UpperSaturationLimit=BLOCKEDTIMER  LowerSaturationLimit=0
  RLServiceEuclideanDistanceCalculator1 : Subsystem
  RLServiceEuclideanDistanceCalculator2 : Subsystem
  Sum : Sum  Inputs=|++
  Sum1 : Sum  Inputs=+-|
  Switch1 : Switch  Criteria=u2 > Threshold  Threshold=0.5
  Switch3 : Switch  Threshold=BLOCKEDTIMER
  Switch4 : Switch  Criteria=u2 > Threshold
  ArrivedCheck : Outport
  wires:
  RLServiceEuclideanDistanceCalculator1/1(DistToGoal) -> Switch1/2
  X/1 -> RLServiceEuclideanDistanceCalculator1/1(X)
  Switch1/1 -> Sum/1
  Constant3/1 -> Switch1/3
  Y/1 -> RLServiceEuclideanDistanceCalculator1/2(Y)
  Constant4/1 -> Switch1/1
  Sum/1 -> ArrivedCheck/1
  Switch3/1 -> Sum/2
  Integrator/1 -> Switch3/2
  Constant5/1 -> Switch3/3
  XRL/1 -> RLServiceEuclideanDistanceCalculator2/1(X)
  YRL/1 -> RLServiceEuclideanDistanceCalculator2/2(Y)
  XGoal/1 -> RLServiceEuclideanDistanceCalculator2/3(GoalX), RLServiceEuclideanDistanceCalculator1/3(GoalX)
  YGoal/1 -> RLServiceEuclideanDistanceCalculator2/4(GoalY), RLServiceEuclideanDistanceCalculator1/4(GoalY)
  RLServiceEuclideanDistanceCalculator2/1(OppDistToGoal) -> Sum1/1
  Constant8/1 -> Switch4/1
  Constant6/1 -> Switch4/3
  THRESHOLD/1 -> Sum1/2
  Sum1/1 -> Switch4/2
  Switch4/1 -> Integrator/1
  Constant1/1 -> Switch3/1

== system RLFactorySensorNoise/RLServiceOpponentB/RLServiceAOpponentController/RLServiceEMAdjustVelocity ==
  DirX : Inport
  DirY : Inport  Port=2
  VIn : Inport  Port=3
  Constant : Constant
  Demux1 : Demux  Outputs=2
  Divide : Product  Inputs=*/
  Divide1 : Product  Inputs=*/
  Mux : Mux  Inputs=2
  Product : Product
  Product3 : Product
  Sqrt1 : Sqrt  SaturateOnIntegerOverflow=on
  Square : Math  Operator=square  SaturateOnIntegerOverflow=on
  Square1 : Math  Operator=square  SaturateOnIntegerOverflow=on
  Sum : Sum  Inputs=+|+
  Switch : Switch  Criteria=u2 > Threshold
  VX : Outport
  VY : Outport  Port=2
  wires:
  Product/1 -> VX/1
  DirY/1 -> Square1/1, Mux/2
  Mux/1 -> Demux1/1
  Divide1/1 -> Product3/1
  Constant/1 -> Switch/3
  Square1/1 -> Sum/2
  Switch/1 -> Divide1/2, Divide/2
  VIn/1 -> Product/2, Product3/2
  Sum/1 -> Sqrt1/1
  Square/1 -> Sum/1
  Sqrt1/1 -> Switch/2, Switch/1
  Product3/1 -> VY/1
  Demux1/2 -> Divide1/1
  DirX/1 -> Square/1, Mux/1
  Demux1/1 -> Divide/1
  Divide/1 -> Product/1

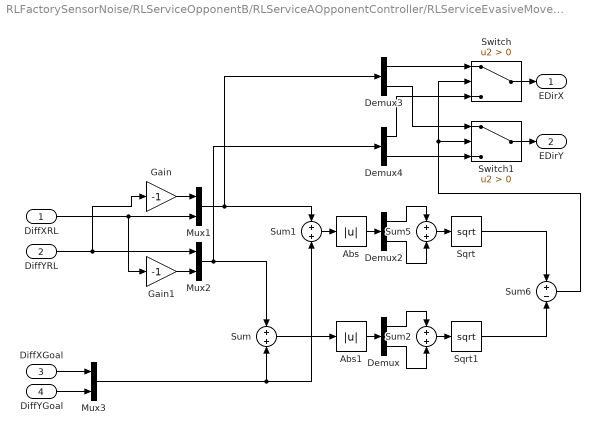
== system RLFactorySensorNoise/RLServiceOpponentB/RLServiceAOpponentController/RLServiceEvasiveMoveChooser ==
  DiffXRL : Inport
  DiffYRL : Inport  Port=2
  DiffXGoal : Inport  Port=3
  DiffYGoal : Inport  Port=4
  Abs : Abs
  Abs1 : Abs
  Demux{,2..4} (4 alike) : Demux  Outputs=2
  Gain : Gain  Gain=-1
  Gain1 : Gain  Gain=-1
  Mux1 : Mux  Inputs=2
  Mux2 : Mux  Inputs=2
  Mux3 : Mux  Inputs=2
  Sqrt : Sqrt  SaturateOnIntegerOverflow=on
  Sqrt1 : Sqrt  SaturateOnIntegerOverflow=on
  Sum{,1..2,5} (4 alike) : Sum  Inputs=+|+
  Sum6 : Sum  Inputs=+|-
  Switch : Switch  Criteria=u2 > Threshold
  Switch1 : Switch  Criteria=u2 > Threshold
  EDirX : Outport
  EDirY : Outport  Port=2
  wires:
  Gain/1 -> Mux1/1
  DiffXRL/1 -> Gain1/1, Mux1/2
  Gain1/1 -> Mux2/2
  DiffXGoal/1 -> Mux3/1
  DiffYGoal/1 -> Mux3/2
  Mux3/1 -> Sum/2, Sum1/2
  Mux2/1 -> Sum/1, Demux4/1
  Mux1/1 -> Demux3/1, Sum1/1
  Sum1/1 -> Abs/1
  Sum/1 -> Abs1/1
  Abs1/1 -> Demux/1
  Demux/1 -> Sum2/1
  Demux/2 -> Sum2/2
  Demux2/2 -> Sum5/2
  Demux2/1 -> Sum5/1
  Abs/1 -> Demux2/1
  Sum5/1 -> Sqrt/1
  Sum2/1 -> Sqrt1/1
  Sqrt/1 -> Sum6/1
  Sqrt1/1 -> Sum6/2
  Sum6/1 -> Switch/2, Switch1/2
  Demux3/1 -> Switch/1
  Demux3/2 -> Switch1/1
  Demux4/1 -> Switch/3
  Demux4/2 -> Switch1/3
  Switch/1 -> EDirX/1
  Switch1/1 -> EDirY/1
  DiffYRL/1 -> Mux2/1, Gain/1

== system RLFactorySensorNoise/RLServiceOpponentB/RLServiceAOpponentController/RLServiceInvalidMoveChecker ==
  VX : Inport
  VY : Inport  Port=2
  DiffXRL : Inport  Port=3
  DiffYRL : Inport  Port=4
  THRESHOLD : Inport  Port=5
  Constant5 : Constant
  Constant6 : Constant  Value=0
  Constant7 : Constant  Value=0
  Constant8 : Constant
  Constant9 : Constant
  Product : Product
  Product1 : Product
  Square : Math  Operator=square  SaturateOnIntegerOverflow=on
  Square Root : Sqrt  SaturateOnIntegerOverflow=on
  Square1 : Math  Operator=square  SaturateOnIntegerOverflow=on
  Sum : Sum  Inputs=+|-
  Sum1 : Sum
  Sum5 : Sum  Inputs=+|+
  Sum6 : Sum  Inputs=+|-|+
  Switch1 : Switch  Criteria=u2 > Threshold
  Switch3 : Switch  Criteria=u2 > Threshold
  MoveInvalid : Outport
  wires:
  Product1/1 -> Sum5/2
  Sum5/1 -> Switch3/2
  Product/1 -> Sum5/1
  Sum6/1 -> MoveInvalid/1
  Switch3/1 -> Sum6/1
  Constant9/1 -> Switch3/1
  VY/1 -> Product1/1
  VX/1 -> Product/1
  Constant8/1 -> Sum6/2
  Constant7/1 -> Switch3/3
  THRESHOLD/1 -> Sum/2
  Sum/1 -> Switch1/2
  Constant5/1 -> Switch1/3
  Constant6/1 -> Switch1/1
  Switch1/1 -> Sum6/3
  DiffYRL/1 -> Square1/1, Product1/2
  DiffXRL/1 -> Product/2, Square/1
  Square1/1 -> Sum1/2
  Sum1/1 -> Square Root/1
  Square/1 -> Sum1/1
  Square Root/1 -> Sum/1

== system RLFactorySensorNoise/RLServiceOpponentB/RLServiceAOpponentController/RLServicePMAdjustVelocity ==
  DirX : Inport
  DirY : Inport  Port=2
  VIn : Inport  Port=3
  Constant : Constant
  Demux1 : Demux  Outputs=2
  Divide : Product  Inputs=*/
  Divide1 : Product  Inputs=*/
  Mux : Mux  Inputs=2
  Product : Product
  Product3 : Product
  Sqrt1 : Sqrt  SaturateOnIntegerOverflow=on
  Square : Math  Operator=square  SaturateOnIntegerOverflow=on
  Square1 : Math  Operator=square  SaturateOnIntegerOverflow=on
  Sum : Sum  Inputs=+|+
  Switch : Switch  Criteria=u2 > Threshold
  VX : Outport
  VY : Outport  Port=2
  wires:
  VIn/1 -> Product/2, Product3/2
  DirX/1 -> Square/1, Mux/1
  DirY/1 -> Square1/1, Mux/2
  Divide1/1 -> Product3/1
  Divide/1 -> Product/1
  Switch/1 -> Divide1/2, Divide/2
  Constant/1 -> Switch/3
  Mux/1 -> Demux1/1
  Demux1/2 -> Divide1/1
  Square1/1 -> Sum/2
  Sum/1 -> Sqrt1/1
  Demux1/1 -> Divide/1
  Product/1 -> VX/1
  Sqrt1/1 -> Switch/2, Switch/1
  Product3/1 -> VY/1
  Square/1 -> Sum/1

== system RLFactorySensorNoise/RLServiceOpponentB/RLServiceAOpponentController/RLServiceXAvoidOvershooting ==
  VX : Inport
  VY : Inport  Port=2
  DiffToGoalX : Inport  Port=3
  DiffToGoalY : Inport  Port=4
  TS : Inport  Port=5
  Abs{1..4} (4 alike) : Abs
  Divide : Product  Inputs=*/
  Divide1 : Product  Inputs=*/
  Product : Product
  Product1 : Product
  Sum1 : Sum  Inputs=-|+
  Sum2 : Sum  Inputs=-|+
  Switch : Switch  Criteria=u2 > Threshold
  Switch1 : Switch  Criteria=u2 > Threshold
  VXNoOvershoot : Outport
  VYNoOvershoot : Outport  Port=2
  wires:
  Abs1/1 -> Sum1/2
  Switch/1 -> VXNoOvershoot/1
  Product/1 -> Abs2/1
  Abs2/1 -> Sum1/1
  DiffToGoalX/1 -> Divide/1, Abs1/1
  Sum1/1 -> Switch/2
  VX/1 -> Product/1, Switch/1
  Divide/1 -> Switch/3
  VY/1 -> Product1/1, Switch1/1
  Sum2/1 -> Switch1/2
  Abs4/1 -> Sum2/1
  Product1/1 -> Abs4/1
  Divide1/1 -> Switch1/3
  TS/1 -> Divide1/2, Product1/2, Divide/2, Product/2
  Abs3/1 -> Sum2/2
  Switch1/1 -> VYNoOvershoot/1
  DiffToGoalY/1 -> Divide1/1, Abs3/1

== system RLFactorySensorNoise/RLServiceRLRobotNoise/RLServiceRLInfo/RLServiceCrashDetector ==
  X : Inport
  Y : Inport  Port=2
  XA : Inport  Port=3
  YA : Inport  Port=4
  XB : Inport  Port=5
  YB : Inport  Port=6
  Constant : Constant  Value=SAFETYDISTANCEA
  Constant1 : Constant  Value=SAFETYDISTANCEB
  Constant2 : Constant  Value=THRESHOLDA
  Constant3 : Constant  Value=THRESHOLDB
  Less Than{1..4} (4 alike) : RelationalOperator  Operator=<=  OutDataTypeStr=boolean  RndMeth=Simplest
  Memory : Memory
  OR : Logic  Operator=OR  IconShape=distinctive  AllPortsSameDT=off  OutDataTypeStr=boolean
  OR1 : Logic  Operator=OR  IconShape=distinctive  AllPortsSameDT=off  OutDataTypeStr=boolean
  RLServiceEuclideanDistanceCalculator1 : Subsystem
  RLServiceEuclideanDistanceCalculator2 : Subsystem
  Switch3 : Switch  Criteria=u2 > Threshold
  BelowThreshold : Outport
  Crash : Outport  Port=2
  wires:
  XA/1 -> RLServiceEuclideanDistanceCalculator1/3(XOpp)
  Less Than2/1 -> OR/1
  Memory/1 -> Switch3/1, Switch3/2
  Constant/1 -> Less Than2/2
  Y/1 -> RLServiceEuclideanDistanceCalculator2/2(Y), RLServiceEuclideanDistanceCalculator1/2(Y)
  YA/1 -> RLServiceEuclideanDistanceCalculator1/4(YOpp)
  X/1 -> RLServiceEuclideanDistanceCalculator1/1(X), RLServiceEuclideanDistanceCalculator2/1(X)
  OR/1 -> Switch3/3
  Constant1/1 -> Less Than3/2
  YB/1 -> RLServiceEuclideanDistanceCalculator2/4(YOpp)
  Less Than3/1 -> OR/2
  XB/1 -> RLServiceEuclideanDistanceCalculator2/3(XOpp)
  Switch3/1 -> Crash/1, Memory/1
  Constant2/1 -> Less Than1/2
  RLServiceEuclideanDistanceCalculator1/1(Dist) -> Less Than2/1, Less Than1/1
  Constant3/1 -> Less Than4/2
  RLServiceEuclideanDistanceCalculator2/1(Dist) -> Less Than4/1, Less Than3/1
  Less Than1/1 -> OR1/1
  Less Than4/1 -> OR1/2
  OR1/1 -> BelowThreshold/1

== system RLFactorySensorNoise/RLServiceRLRobotNoise/RLServiceRLInfo/RLServiceGoalTracker ==
  X : Inport
  Y : Inport  Port=2
  XGoal : Inport  Port=3
  YGoal : Inport  Port=4
  Constant1 : Constant
  Constant5 : Constant  Value=0.5
  Constant7 : Constant  Value=0
  Less Than1 : RelationalOperator  Operator=<  OutDataTypeStr=boolean  RndMeth=Simplest
  RLServiceEuclideanDistanceCalculator : Subsystem
  Switch : Switch  Criteria=u2 > Threshold
  Dist : Outport
  Arrived : Outport  Port=2
  wires:
  Constant7/1 -> Switch/3
  XGoal/1 -> RLServiceEuclideanDistanceCalculator/3(GoalX)
  Y/1 -> RLServiceEuclideanDistanceCalculator/2(Y)
  RLServiceEuclideanDistanceCalculator/1(DistGoal) -> Dist/1, Less Than1/1
  Constant1/1 -> Switch/1
  Switch/1 -> Arrived/1
  Less Than1/1 -> Switch/2
  X/1 -> RLServiceEuclideanDistanceCalculator/1(X)
  YGoal/1 -> RLServiceEuclideanDistanceCalculator/4(GoalY)
  Constant5/1 -> Less Than1/2

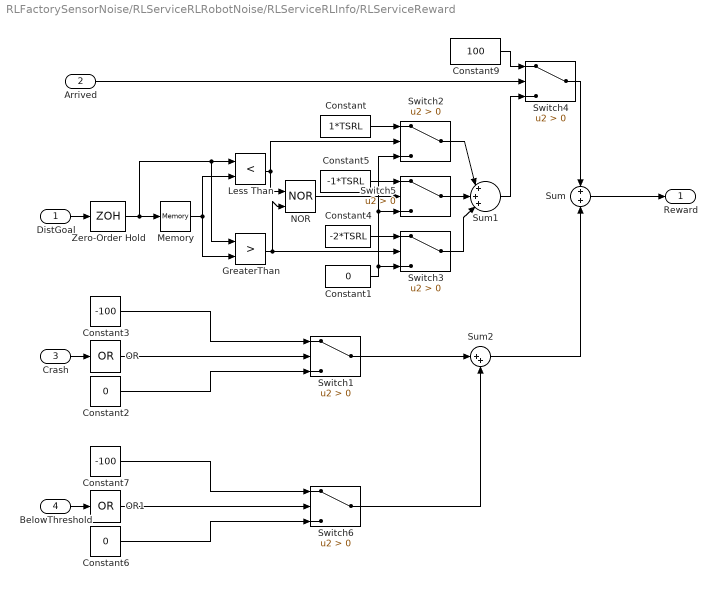
== system RLFactorySensorNoise/RLServiceRLRobotNoise/RLServiceRLInfo/RLServiceReward ==
  DistGoal : Inport
  Arrived : Inport  Port=2
  Crash : Inport  Port=3
  BelowThreshold : Inport  Port=4
  Constant : Constant  Value=1*TSRL
  Constant1 : Constant  Value=0
  Constant2 : Constant  Value=0
  Constant3 : Constant  Value=-100  VectorParams1D=off
  Constant4 : Constant  Value=-2*TSRL
  Constant5 : Constant  Value=-1*TSRL
  Constant6 : Constant  Value=0
  Constant7 : Constant  Value=-100  VectorParams1D=off
  Constant9 : Constant  Value=100
  GreaterThan : RelationalOperator  Operator=>  OutDataTypeStr=boolean  RndMeth=Simplest
  Less Than : RelationalOperator  Operator=<  OutDataTypeStr=boolean  RndMeth=Simplest
  Memory : Memory
  NOR : Logic  Operator=NOR  IconShape=distinctive  AllPortsSameDT=off  OutDataTypeStr=boolean
  OR : Logic  Operator=OR  Inputs=1  IconShape=distinctive  AllPortsSameDT=off  OutDataTypeStr=boolean
  OR1 : Logic  Operator=OR  Inputs=1  IconShape=distinctive  AllPortsSameDT=off  OutDataTypeStr=boolean
  Sum : Sum
  Sum1 : Sum  Inputs=|+++|
  Sum2 : Sum  Inputs=|++
  Switch{1..6} (6 alike) : Switch  Criteria=u2 > Threshold
  Zero-Order Hold : ZeroOrderHold  SampleTime=TSRL
  Reward : Outport
  wires:
  Sum/1 -> Reward/1
  Constant2/1 -> Switch1/3
  Constant3/1 -> Switch1/1
  Sum2/1 -> Sum/2
  DistGoal/1 -> Zero-Order Hold/1
  Memory/1 -> GreaterThan/2, Less Than/2
  Switch4/1 -> Sum/1
  Constant9/1 -> Switch4/1
  Switch2/1 -> Sum1/1
  Arrived/1 -> Switch4/2
  OR/1 -> Switch1/2
  Less Than/1 -> NOR/1, Switch2/2
  Constant/1 -> Switch2/1
  Constant1/1 -> Switch2/3, Switch5/3, Switch3/3
  GreaterThan/1 -> NOR/2, Switch3/2
  Constant4/1 -> Switch3/1
  Sum1/1 -> Switch4/3
  Switch3/1 -> Sum1/3
  NOR/1 -> Switch5/2
  Constant5/1 -> Switch5/1
  Switch5/1 -> Sum1/2
  Zero-Order Hold/1 -> Memory/1, GreaterThan/1, Less Than/1
  Crash/1 -> OR/1
  OR1/1 -> Switch6/2
  Constant7/1 -> Switch6/1
  BelowThreshold/1 -> OR1/1
  Constant6/1 -> Switch6/3
  Switch6/1 -> Sum2/2
  Switch1/1 -> Sum2/1

== system RLFactorySensorNoise/RLServiceRLRobotNoise/RLServiceRLMotorControl/RLServiceRLAdjustVelocity ==
  DirX : Inport
  DirY : Inport  Port=2
  VIn : Inport  Port=3
  Constant : Constant
  Demux1 : Demux  Outputs=2
  Divide : Product  Inputs=*/
  Divide1 : Product  Inputs=*/
  Mux : Mux  Inputs=2
  Product : Product
  Product3 : Product
  Sqrt1 : Sqrt  SaturateOnIntegerOverflow=on
  Square : Math  Operator=square  SaturateOnIntegerOverflow=on
  Square1 : Math  Operator=square  SaturateOnIntegerOverflow=on
  Sum : Sum  Inputs=+|+
  Switch : Switch  Criteria=u2 > Threshold
  VX : Outport
  VY : Outport  Port=2
  wires:
  Product/1 -> VX/1
  DirY/1 -> Square1/1, Mux/2
  Mux/1 -> Demux1/1
  Divide1/1 -> Product3/1
  Constant/1 -> Switch/3
  Square1/1 -> Sum/2
  Switch/1 -> Divide1/2, Divide/2
  VIn/1 -> Product/2, Product3/2
  Sum/1 -> Sqrt1/1
  Square/1 -> Sum/1
  Sqrt1/1 -> Switch/2, Switch/1
  Product3/1 -> VY/1
  Demux1/2 -> Divide1/1
  DirX/1 -> Square/1, Mux/1
  Demux1/1 -> Divide/1
  Divide/1 -> Product/1

== system RLFactorySensorNoise/RLServiceRLRobotNoise/RLServiceRLRobotSensorWithDMAXAndNoise/RLServiceARobotSensorSubsystemWithDMAXAndNoise ==
  XRL : Inport
  YRL : Inport  Port=2
  XOpp : Inport  Port=3
  YOpp : Inport  Port=4
  Constant : Constant  Value=0
  Constant1 : Constant  Value=DMAX
  Product : Product
  Product1 : Product
  RLServiceNoise : Subsystem
  RLServiceRobotSensorSubsystem : Subsystem
  Sqrt1 : Sqrt  SaturateOnIntegerOverflow=on
  Square : Math  Operator=square  SaturateOnIntegerOverflow=on
  Square1 : Math  Operator=square  SaturateOnIntegerOverflow=on
  Sum1 : Sum  Inputs=+|+
  Switch{,1..3} (4 alike) : Switch  Criteria=u2 > Threshold  Threshold=CUTOFF
  DiffX : Outport
  DiffY : Outport  Port=2
  DirX : Outport  Port=3
  DirY : Outport  Port=4
  wires:
  Switch1/1 -> DirY/1
  Constant1/1 -> Switch2/1
  Product1/1 -> Switch2/3, Square1/1
  RLServiceRobotSensorSubsystem/4(DirYOpp) -> Switch1/3
  Constant/1 -> Switch/1, Switch3/1, Switch1/1
  Sum1/1 -> Sqrt1/1
  YOpp/1 -> RLServiceRobotSensorSubsystem/4(YOpp)
  XOpp/1 -> RLServiceRobotSensorSubsystem/3(XOpp)
  Switch/1 -> DirX/1
  RLServiceNoise/1(Out1) -> Product1/1, Product/1
  Square1/1 -> Sum1/2
  Switch3/1 -> DiffX/1
  Sqrt1/1 -> Switch1/2, Switch/2, Switch2/2, Switch3/2
  XRL/1 -> RLServiceRobotSensorSubsystem/1(X)
  YRL/1 -> RLServiceRobotSensorSubsystem/2(Y)
  RLServiceRobotSensorSubsystem/3(DirXOpp) -> Switch/3
  Switch2/1 -> DiffY/1
  RLServiceRobotSensorSubsystem/1(DiffXOpp) -> Product/2
  RLServiceRobotSensorSubsystem/2(DiffYOpp) -> Product1/2
  Square/1 -> Sum1/1
  Product/1 -> Switch3/3, Square/1

== system RLFactorySensorNoise/RLServiceRLRobotNoise/RLServiceRLRobotSensorWithDMAXAndNoise/RLServiceBRobotSensorSubsystemWithDMAXAndNoise ==
  XRL : Inport
  YRL : Inport  Port=2
  XOpp : Inport  Port=3
  YOpp : Inport  Port=4
  Constant : Constant  Value=0
  Constant1 : Constant  Value=DMAX
  Product : Product
  Product1 : Product
  RLServiceNoise : Subsystem
  RLServiceRobotSensorSubsystem : Subsystem
  Sqrt1 : Sqrt  SaturateOnIntegerOverflow=on
  Square : Math  Operator=square  SaturateOnIntegerOverflow=on
  Square1 : Math  Operator=square  SaturateOnIntegerOverflow=on
  Sum1 : Sum  Inputs=+|+
  Switch{,1..3} (4 alike) : Switch  Criteria=u2 > Threshold  Threshold=CUTOFF
  DiffX : Outport
  DiffY : Outport  Port=2
  DirX : Outport  Port=3
  DirY : Outport  Port=4
  wires:
  Product/1 -> Square/1, Switch3/3
  Square/1 -> Sum1/1
  RLServiceRobotSensorSubsystem/2(DiffOppY) -> Product1/2
  RLServiceRobotSensorSubsystem/1(DiffOppX) -> Product/2
  Switch2/1 -> DiffY/1
  RLServiceRobotSensorSubsystem/3(DirOppX) -> Switch/3
  YRL/1 -> RLServiceRobotSensorSubsystem/2(Y)
  XRL/1 -> RLServiceRobotSensorSubsystem/1(X)
  Sqrt1/1 -> Switch3/2, Switch2/2, Switch/2, Switch1/2
  Switch3/1 -> DiffX/1
  Square1/1 -> Sum1/2
  RLServiceNoise/1(Out1) -> Product/1, Product1/1
  Switch/1 -> DirX/1
  XOpp/1 -> RLServiceRobotSensorSubsystem/3(XOpp)
  YOpp/1 -> RLServiceRobotSensorSubsystem/4(YOpp)
  Sum1/1 -> Sqrt1/1
  Constant/1 -> Switch1/1, Switch3/1, Switch/1
  RLServiceRobotSensorSubsystem/4(DirOppY) -> Switch1/3
  Product1/1 -> Square1/1, Switch2/3
  Constant1/1 -> Switch2/1
  Switch1/1 -> DirY/1

== system RLFactorySensorNoise/RLServiceOpponentA/RLServiceAOpponentController/RLServiceArrivedChecker/RLServiceEuclideanDistanceCalculator1 ==
  X : Inport
  Y : Inport  Port=2
  GoalX : Inport  Port=3
  GoalY : Inport  Port=4
  Square : Math  Operator=square  SaturateOnIntegerOverflow=on
  Square Root : Sqrt  SaturateOnIntegerOverflow=on
  Square1 : Math  Operator=square  SaturateOnIntegerOverflow=on
  Sum1 : Sum
  Sum3 : Sum  Inputs=+-
  Sum4 : Sum  Inputs=+-
  DistToGoal : Outport
  wires:
  GoalX/1 -> Sum3/2
  X/1 -> Sum3/1
  Sum1/1 -> Square Root/1
  Sum4/1 -> Square1/1
  Square/1 -> Sum1/1
  Y/1 -> Sum4/1
  Square Root/1 -> DistToGoal/1
  Square1/1 -> Sum1/2
  Sum3/1 -> Square/1
  GoalY/1 -> Sum4/2

== system RLFactorySensorNoise/RLServiceOpponentA/RLServiceAOpponentController/RLServiceArrivedChecker/RLServiceEuclideanDistanceCalculator2 ==
  X : Inport
  Y : Inport  Port=2
  GoalX : Inport  Port=3
  GoalY : Inport  Port=4
  Square : Math  Operator=square  SaturateOnIntegerOverflow=on
  Square Root : Sqrt  SaturateOnIntegerOverflow=on
  Square1 : Math  Operator=square  SaturateOnIntegerOverflow=on
  Sum1 : Sum
  Sum3 : Sum  Inputs=+-
  Sum4 : Sum  Inputs=+-
  OppDistToGoal : Outport
  wires:
  GoalX/1 -> Sum3/2
  X/1 -> Sum3/1
  Sum1/1 -> Square Root/1
  Sum4/1 -> Square1/1
  Square/1 -> Sum1/1
  Y/1 -> Sum4/1
  Square Root/1 -> OppDistToGoal/1
  Square1/1 -> Sum1/2
  Sum3/1 -> Square/1
  GoalY/1 -> Sum4/2

== system RLFactorySensorNoise/RLServiceOpponentB/RLServiceAOpponentController/RLServiceArrivedChecker/RLServiceEuclideanDistanceCalculator1 ==
  X : Inport
  Y : Inport  Port=2
  GoalX : Inport  Port=3
  GoalY : Inport  Port=4
  Square : Math  Operator=square  SaturateOnIntegerOverflow=on
  Square Root : Sqrt  SaturateOnIntegerOverflow=on
  Square1 : Math  Operator=square  SaturateOnIntegerOverflow=on
  Sum1 : Sum
  Sum3 : Sum  Inputs=+-
  Sum4 : Sum  Inputs=+-
  DistToGoal : Outport
  wires:
  GoalX/1 -> Sum3/2
  X/1 -> Sum3/1
  Sum1/1 -> Square Root/1
  Sum4/1 -> Square1/1
  Square/1 -> Sum1/1
  Y/1 -> Sum4/1
  Square Root/1 -> DistToGoal/1
  Square1/1 -> Sum1/2
  Sum3/1 -> Square/1
  GoalY/1 -> Sum4/2
